simulink model "Wall_Model_Version_1_8_2018a"  (R2018b)
settings: Solver=ode3  StartTime=0.0  StopTime=inf  FixedStep=Ts  RelTol=1e-3  EnableMultiTasking=on
InitFcn:
  | clc;
  | clear all;
  | close all;
  | addpath('D:\Aravind_A0164966M_EE5003\Matlab files\3r2c model')
  | Ts=1
  | Duration=36000;
  | %% Coefficients of Rs and Cs
  | 
  | %% Front Wall
  | l1 = 7.37;
  | b1 = 2.63;
  | y1 = 0.186;
  | x1 = 0.111;
  | y2 = 0.814;
  | x2 = 0.506;
  | x3 = 0.383;
  | 
  | %% Left Wall
  | l2 = 10.11;
  | b2 = 2.63;
  | y3 = 0.186;
  | x4 = 0.111;
  | y4 = 0.814;
  | x5 = 0.506;
  | x6 = 0.383;
  | 
  | %% Left Wall Glass
  | x4_g = 0.5;
  | x5_g = 0.5;
  | y3_g = 1;
  | 
  | %% Right Wall
  | l3 = 7.37;
  | b3 = 2.63;
  | y5 = 0.186;
  | x7 = 0.111;
  | y6 = 0.814;
  | x8 = 0.506;
  | x9 = 0.383;
  | 
  | %% Back Wall
  | l4 = 10.11;
  | b4 = 2.63;
  | y7 = 1;
  | x10 = 0.5;
  | %y8 = 0.5;
  | x11 = 0.5;
  | %x12= 0.33;
  | 
  | %% Roof
  | l5 = 10.11;
  | b5 = 7.37;
  | y9 = 0.186;
  | x13 = 0.111;
  | y10 = 0.814;
  | x14 = 0.506;
  | x15 = 0.383;
  | 
  | %% Floor
  | l6 = 10.11;
  | b6 = 7.37;
  | y11 = 0.186;
  | x16 = 0.111;
  | y12 = 0.814;
  | x17 = 0.506;
  | x18 = 0.383;
  | 
  | %%Areas
  | A1 = l1 * b1;
  | A2 = l2 * b2;
  | A3 = l3 * b3;
  | A4 = l4 * b4;
  | A5 = l5 * b5;
  | A6 = l6 * b6;
  | 
  | %% Initial Temperatures at the surfaces
  | T1_initial_front=301;
  | T2_initial_front=300;
  | 
  | T1_initial_left=301;
  | T2_initial_left=300;
  | 
  | T1_initial_right=301;
  | T2_initial_right=300;
  | 
  | T1_initial_back=301;
  | T2_initial_back=300;
  | 
  | T1_initial_roof=301;
  | T2_initial_roof=300;
  | 
  | T1_initial_floor=301;
  | T2_initial_floor=300;
  | 
  | %ri = 0.1300; % m2 K/W resistance of inner surface of brick wall
  | %rso = 0.04; % m2 K/W resistance of outer surface of the wall
  | 
  | ri = 0;
  | rso = 0;
  | %% Density of Building materials in the room
  | p_conc    = 2400; % kg/m3 density of concrete
  | p_pstr     = 850; % kg/m3 density of plastering
  | p_gb       = 1100; % kg/m3 density of gypsum board
  | p_glass    = 2530; % kg/m3 density of glass
  | p_swood  = 550;   % kg/m3 density of soft-wood
  | 
  | %% Thermal heat capacity of the building materials in the room
  | c_conc    = 840;  % J/kg K heat capacity of concrete
  | c_pstr     = 1000;  %J/kg K heat capacity of plastering
  | c_gb       = 700; % J/kg K heat capacity of gypsum board
  | c_glass    = 840;  % J/kg K heat capacity of glass
  | c_swood  = 1700; % J/kg K heat capacity of soft-wood
  | 
  | %% Thermal conductivity(lamda) of building materials in the room
  | l_conc    = 0.8;  % W/m K Thermal conductivity of concrete
  | l_pstr     = 0.013;  % W/m K Thermal conductivity of plastering
  | l_gb       = 0.35; % W/m K Thermal conductivity of gypsum board
  | l_glass    = 0.8;  % W/m K Thermal conductivity of glass
  | l_swood  = 0.08; % W/m K Thermal conductivity of soft-wood
  | 
  | %% Standard thickness of materials used
  | d_conc = 0.01;  % m Thickness of concrete BCA standard
  | d_pstr = 0.005; % m Thickness of plastering BCA standard
  | d_glass = 0.015; % m Thickness of glass wall widely used
  | d_swood = 0.01; % m Thickness of softwood on the right wall
  | d_gb = 0.015; % m Thickness of gypsum board
  | 
  | %% Resistance and Capacitance of front Wall
  | Rth1 =( ri + rso + (d_conc/l_conc) + (d_pstr/l_pstr))/(A1); % Thermal resistance
  | Cth1 = A1*(d_conc*p_conc*c_conc + d_pstr*p_pstr*c_pstr) ; % Thermal Capacitance
  | 
  | %% Resistance and Capacitance of left Wall concrete
  | A_conc = A2 * 0.5; % Half of the wall on the left is  glass wall
  | Rth2 =( ri + rso + (d_conc/l_conc) + (d_pstr/l_pstr))/(A_conc); % Thermal resistance
  | Cth2 = A_conc*(d_conc*p_conc*c_conc + d_pstr*p_pstr*c_pstr); % Thermal Capacitance
  | 
  | %% Resistance and Capacitance of left Wall glass
  | A_glass = A2 * 0.5; % Half of the wall on the left is  glass wall
  | Rth2_g =(d_glass/l_glass) /(A_glass); % Thermal resistance
  | Cth2_g = A_glass*(d_glass*p_glass*c_glass ); % Thermal Capacitance
  | 
  | %% Resistance and Capacitance of right Wall
  | Rth3 = ( ri + rso+ (d_conc/l_conc) + (d_swood/l_swood))/(A3);% Thermal resistance
  | Cth3 = A3*(d_swood*p_swood*c_swood + d_conc*p_conc*c_conc ); % Thermal Capacitance
  | 
  | %% Resistance and Capacitance of back Wall
  | Rth4 =(d_glass/l_glass) /(A4); % Thermal resistance
  | Cth4 = A4*(d_glass*p_glass*c_glass ); % Thermal Capacitance
  | 
  | %% Resistance and Capacitance of roof Wall
  | Rth5 = (d_gb/l_gb)/(A5);% Thermal resistance
  | Cth5 = A5*(d_gb*p_gb*c_gb ); % Thermal Capacitance
  | 
  | %% Resistance and Capacitance of floor Wall
  | Rth6 = (d_gb/l_gb)/(A6);% Thermal resistance
  | Cth6 = A6*(d_gb*p_gb*c_gb ); % Thermal Capacitance
  | 
  | %% Volume and mass of room
  | density_of_air = 1.184; % kg/m3 at 25 deg. K
  | volume = l1*l2*b1; % m3
  | mass = volume * density_of_air ;% kg
  | specific_heat = 1.005; % J/kg deg.K
  | tic;
  | 
  | Tleft = 298;
libraries: powerlib x70, simulink x1
(part 1 of 2)
settings Model: EnablePacing=on  PacingRate=1000  Creator=elekkr  LastModifiedBy=accma
settings DataIOCC: LimitDataPoints=on  SaveFormat=Array
settings OptimizationCC: LifeSpan=inf
settings DebuggingCC: UnconnectedInputMsg=none  UnconnectedOutputMsg=none  UnconnectedLineMsg=none  LibraryContextMissingDiagnostic=none  SFUnexpectedBacktrackingDiag=warning  SFNoUnconditionalDefaultTransitionDiag=warning  SFExecutionAtInitializationDiag=none
settings HardwareCC: ProdBitPerPointer=32  ProdBitPerSizeT=32  ProdBitPerPtrDiffT=32  ProdLargestAtomicFloat=None  ProdIntDivRoundTo=Undefined  ProdEndianess=Unspecified  ProdWordSize=32  ProdHWDeviceType=32-bit Generic
settings ModelReferenceCC: PropagateSignalLabelsOutOfModel=off
settings SFSimCC: SimUseLocalCustomCode=off
settings RTWCC: RTWUseLocalCustomCode=off
settings CodeAppCC: StateflowObjectComments=on
settings GRTTargetCC: TargetLangStandard=C89/C90 (ANSI)  GeneratePreprocessorConditionals=Disable all
settings ConfigComp: CovMetricSettings=dw  CovHtmlReporting=on  CovSaveCumulativeToWorkspaceVar=on  CovSaveSingleToWorkspaceVar=on  CovExternalEMLEnable=off
settings SimscapeCC: SimscapeNormalizeSystem=off

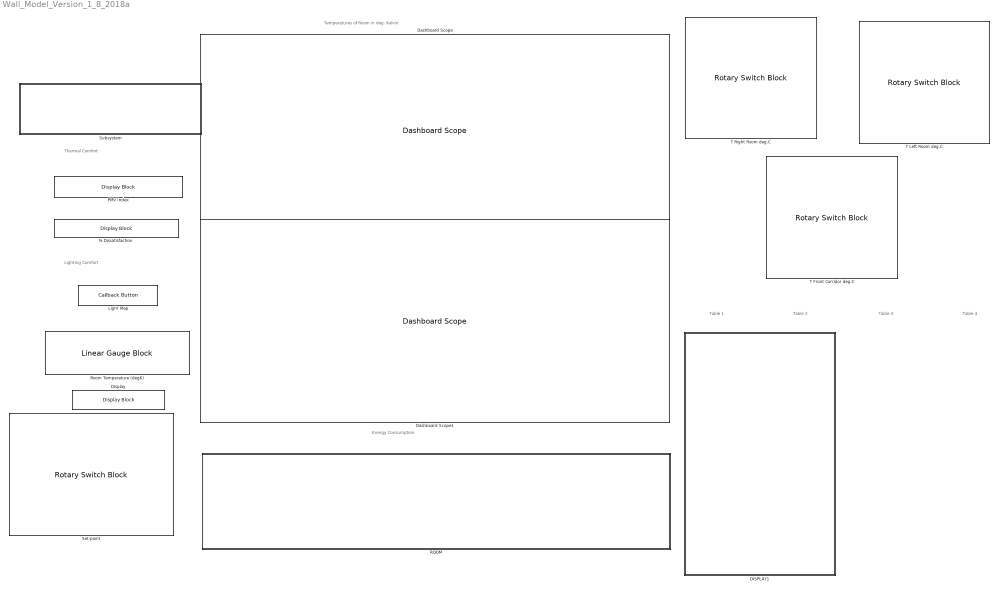
== system Wall_Model_Version_1_8_2018a ==
  note: Table 1
  note: Thermal Comfort
  note: Lighting Comfort
  note: Temperatures of Room in deg. Kelvin
  note: Energy Consumption
  note: Table 2
  note: Table 3
  note: Table 4
  % Dissatisfaction : DisplayBlock  WebBlockId=889  LabelPosition=Hide
  DISPLAY1 : Subsystem  mask(Sensor_node){}
      mask Display: fprintf('CO2 889.35 ppm\n\nCO 1.00 ppm\n\nHCHO 0.03 ppm\n\nO3 0.50 ppm\n\nVOC 0.31 ppm\n\nPM2_5 0.50 ppm\n\nPM10 0.50 ppm\n\nAir Quality Index 82.03\n\n')
  Dashboard Scope : DashboardScope  WebBlockId=1753  Ymin=270  Ymax=330
  Dashboard Scope1 : DashboardScope  WebBlockId=1752  Ymin=0  Ymax=10000
  Display : DisplayBlock  WebBlockId=772  LabelPosition=Hide
  Light Map : CallbackButton  WebBlockId=904
      settings: ClickFcn=heatmap_V2
  PMV Index : DisplayBlock  WebBlockId=888  LabelPosition=Hide
  ROOM : Subsystem
  Room Temperature (degK) : LinearGaugeBlock  WebBlockId=1755  ScaleMin=20  ScaleMax=29  TickInterval=5
  Set-point : RotarySwitchBlock  WebBlockId=542  LabelPosition=Hide
      settings: Values={{'Cold', '', '', 'Optimum', '', '', '', '', '', '', 'Hot'}, [293 294 295 296 297 298 299 300 301 302 303]}
  Subsystem : Subsystem  mask(GBIC_Simulation time){}
      settings: AttributesFormatString=311.25
      mask Display: fprintf('Simulation_Time_Elapsed=1387.00 seconds\nPhysical_Time_Elapsed=311.25 seconds\nSimulation_Speed=4.46 times')
  T Front Corridor deg.C : RotarySwitchBlock  WebBlockId=766  LabelPosition=Hide
      settings: Values={{'20', '21', '22', '23', '24', '25', '26', '27', '28', '29', '30', '31', '32'}, [293 294 295 296 297 298 299 300 301 302 303 304 305]}
  T Left Room deg.C : RotarySwitchBlock  WebBlockId=768  LabelPosition=Hide
      settings: Values={{'20', '21', '22', '23', '24', '25', '26', '27', '28', '29', '30', '31', '32'}, [293 294 295 296 297 298 299 300 301 302 303 304 305]}
  T Right Room deg.C : RotarySwitchBlock  WebBlockId=769  LabelPosition=Hide
      settings: Values={{'20', '21', '22', '23', '24', '25', '26', '27', '28', '29', '30', '31', '32'}, [293 294 295 296 297 298 299 300 301 302 303 304 305]}

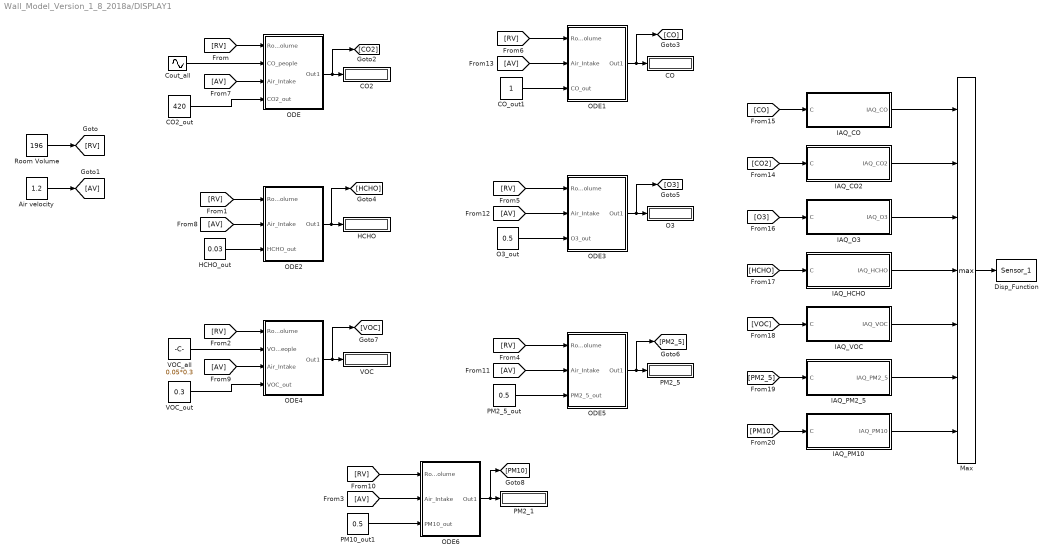
== system Wall_Model_Version_1_8_2018a/DISPLAY1 ==
  Air velocity : Constant  Value=1.2
  CO : Display
  CO2 : Display
  CO2_out : Constant  Value=420
  CO_out1 : Constant
  Cout_all : Sin  Amplitude=150  Bias=550  Frequency=2*pi/(24*3600)
  Disp_Function : M-S-Function  FunctionName=Sensor_1
  HCHO : Display
  HCHO_out : Constant  Value=0.03
  IAQ_CO : MATLAB Function  TreatAsAtomicUnit=on
  IAQ_CO2 : MATLAB Function  TreatAsAtomicUnit=on
  IAQ_HCHO : MATLAB Function  TreatAsAtomicUnit=on
  IAQ_O3 : MATLAB Function  TreatAsAtomicUnit=on
  IAQ_PM10 : MATLAB Function  TreatAsAtomicUnit=on
  IAQ_PM2_5 : MATLAB Function  TreatAsAtomicUnit=on
  IAQ_VOC : MATLAB Function  TreatAsAtomicUnit=on
  Max : MinMax  Function=max  Inputs=7
  O3 : Display
  O3_out : Constant  Value=0.5
  ODE : Subsystem
  ODE1 : Subsystem
  ODE2 : Subsystem
  ODE3 : Subsystem
  ODE4 : Subsystem
  ODE5 : Subsystem
  ODE6 : Subsystem
  PM10_out1 : Constant  Value=0.5
  PM2_1 : Display
  PM2_5 : Display
  PM2_5_out : Constant  Value=0.5
  Room Volume : Constant  Value=196
  VOC : Display
  VOC_all : Constant  Value=0.05*0.3
  VOC_out : Constant  Value=0.3
  wires:
  Cout_all/1 -> ODE/2(CO_people)
  ODE2/1(Out1) -> [HCHO], HCHO/1
  HCHO_out/1 -> ODE2/3(HCHO_out)
  CO_out1/1 -> ODE1/3(CO_out)
  CO2_out/1 -> ODE/4(CO2_out)
  O3_out/1 -> ODE3/3(O3_out)
  ODE3/1(Out1) -> [O3], O3/1
  IAQ_CO/1(IAQ_CO) -> Max/1
  IAQ_HCHO/1(IAQ_HCHO) -> Max/4
  ODE/1(Out1) -> [CO2], CO2/1
  IAQ_CO2/1(IAQ_CO2) -> Max/2
  IAQ_PM2_5/1(IAQ_PM2_5) -> Max/6
  IAQ_VOC/1(IAQ_VOC) -> Max/5
  IAQ_PM10/1(IAQ_PM10) -> Max/7
  ODE1/1(Out1) -> [CO], CO/1
  IAQ_O3/1(IAQ_O3) -> Max/3
  ODE5/1(Out1) -> [PM2_5], PM2_5/1
  PM2_5_out/1 -> ODE5/3(PM2_5_out)
  Room Volume/1 -> [RV]
  [RV] -> ODE/1(Room_Volume)
  [RV] -> ODE2/1(Room_Volume)
  [RV] -> ODE5/1(Room_Volume)
  [RV] -> ODE3/1(Room_Volume)
  [RV] -> ODE1/1(Room_Volume)
  Air velocity/1 -> [AV]
  [AV] -> ODE/3(Air_Intake)
  [AV] -> ODE2/2(Air_Intake)
  [AV] -> ODE5/2(Air_Intake)
  [AV] -> ODE3/2(Air_Intake)
  [AV] -> ODE1/2(Air_Intake)
  [RV] -> ODE4/1(Room_Volume)
  ODE4/1(Out1) -> [VOC], VOC/1
  [AV] -> ODE4/3(Air_Intake)
  VOC_out/1 -> ODE4/4(VOC_out)
  VOC_all/1 -> ODE4/2(VOC_people)
  [AV] -> ODE6/2(Air_Intake)
  [RV] -> ODE6/1(Room_Volume)
  PM10_out1/1 -> ODE6/3(PM10_out)
  [CO2] -> IAQ_CO2/1(C)
  [CO] -> IAQ_CO/1(C)
  [O3] -> IAQ_O3/1(C)
  [HCHO] -> IAQ_HCHO/1(C)
  [VOC] -> IAQ_VOC/1(C)
  [PM2_5] -> IAQ_PM2_5/1(C)
  [PM10] -> IAQ_PM10/1(C)
  ODE6/1(Out1) -> [PM10], PM2_1/1
  Max/1 -> Disp_Function/1

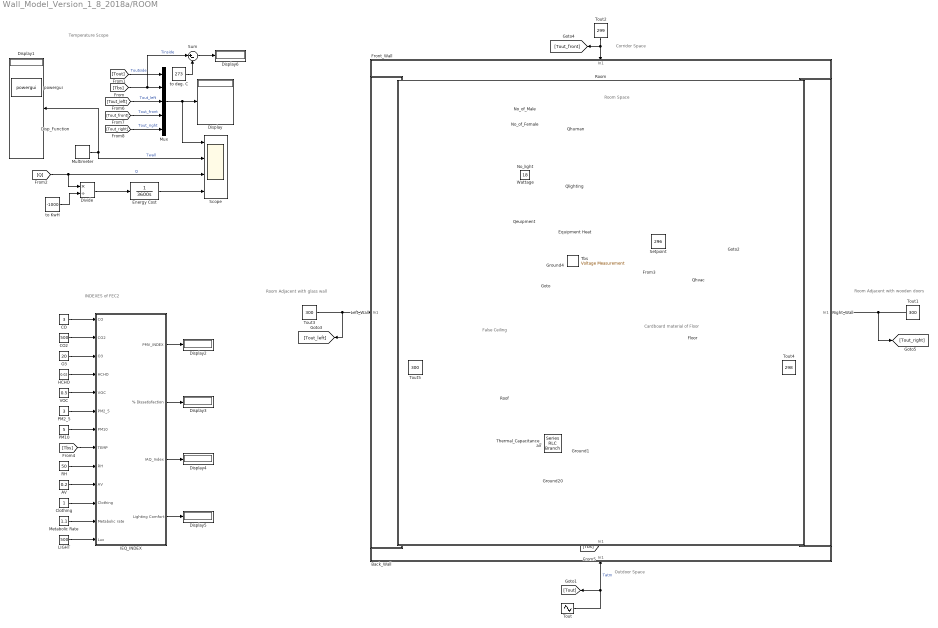
== system Wall_Model_Version_1_8_2018a/ROOM ==
  note: INDEXES of FEC2
  note: False Ceiling
  note: Cardboard material of Floor
  note: Room Adjacent with wooden doors
  note: Corridor Space
  note: Room Adjacent with glass wall
  note: Outdoor Space
  note: Room Space
  note: Temperature Scope
  AV : Constant  Value=0.2
  Back_Wall : Subsystem
      mask Display: fprintf('Temperature Outside= 30.30 deg. C\n')
  CO : Constant  Value=3
  CO2 : Constant  Value=500
  Clothing : Constant
  Disp_Function : M-S-Function  FunctionName=fn_IEQ
  Display{,1..6} (7 alike) : Display
  Divide : Product  Inputs=*/
  Energy Cost : TransferFcn  Denominator=[3600 0]
  Equipment Heat : Subsystem
  Floor : Subsystem
      mask Display: fprintf('Temperature \n Below= \n25.00 deg. C\n')
  Front_Wall : Subsystem
      mask Display: fprintf('Temperature Corridor= 26.00 deg. C\n')
  Ground1 : powerlib/Elements/Ground  LConnTagsString=a
      settings: SourceProductName=Simscape Electrical
  Ground20 : powerlib/Elements/Ground  LConnTagsString=a
      settings: SourceProductName=Simscape Electrical
  Ground4 : powerlib/Elements/Ground  LConnTagsString=a
      settings: SourceProductName=Simscape Electrical
  HCHO : Constant  Value=0.02
  IEQ_INDEX : Subsystem
  LIGHT : Constant  Value=500
  Left_Wall : Subsystem
      mask Display: fprintf('Temperature \n Left Room= \n27.00 deg. C\n')
  Metabolic Rate : Constant  Value=1.1
  Multimeter : powerlib/Measurements/Multimeter  PhasorSimulation=off  OutputType=Complex  sel=1  L=12  Gain=0  yselected={}  PSBOutputType=1  PSBequivalent=0  AxesSetting=[0,0.1,-100,100]  Display=0  SavedBlockNames=-11
      settings: SourceProductName=Simscape Electrical
  Mux : Mux  Inputs=5
  No_light : Constant  Value=60
  No_of_Female : Constant  Value=8
  No_of_Male : Constant  Value=8
  O3 : Constant  Value=20
  PM10 : Constant  Value=5
  PM2_5 : Constant  Value=3
  Qeuipment : Sin  Amplitude=200  Bias=3200  Frequency=2*pi/(12*3600)  SampleTime=0
  Qhuman : Subsystem
  Qhvac : Subsystem
  Qlighting : Subsystem
  RH : Constant  Value=50
  Right_Wall : Subsystem
      mask Display: fprintf('Temperature \n Right Room= \n27.00 deg. C\n')
  Roof : Subsystem
      mask Display: fprintf('Temperature \n Above Roof= \n27.00 deg. C\n')
  Room : Subsystem
      mask Display: fprintf('Temperature Room= 23.00 deg. C\n')
  Scope : Scope  NumInputPorts=4
  Setpoint : Constant  Value=296
  Sum : Sum  Inputs=|+-
  Tbs : powerlib/Measurements/Voltage Measurement  PhasorSimulation=off  OutputType=Magnitude  PSBequivalent=0
      settings: SourceProductName=Simscape Electrical
  Thermal_Capacitance_air : powerlib/Elements/Series RLC Branch  LConnTagsString=__new0  RConnTagsString=__new0  BranchType=C  Resistance=0  Inductance=1e-3  SetiL0=off  InitialCurrent=0  Capacitance=density_of_air * volume * specific_heat  Setx0=on  InitialVoltage=298  Measurements=Branch voltage
      settings: SourceProductName=Simscape Electrical
  Tout : Sin  Amplitude=1.5  Bias=303  Frequency=2*pi/(12*3600)
  Tout1 : Constant  Value=300
  Tout2 : Constant  Value=299
  Tout3 : Constant  Value=300
  Tout4 : Constant  Value=298
  Tout5 : Constant  Value=300
  VOC : Constant  Value=0.5
  Wattage : Constant  Value=18
  powergui : powerlib/powergui  Priority=1  SimulationMode=Discrete  SampleTime=Ts  frequency=60  Iterations=50  frequencyindice=0  Pbase=100e6  ErrMax=1e-4  UnitsV=kV  UnitsW=MW  buscounter=0  FunctionMessages=off  echomessages=off  EnableUseOfTLC=off  CurrentSourceSwitches=off  DisableSnubberDevices=off  DisableRonSwitches=off  DisableVfSwitches=off  DisplayEquations=off  SolverType=Tustin/Backward Euler (TBE)  Interpol=off  ExternalGateDelay=off  methode=off  Ts=100  x0status=blocks  SPID=off  SwTol=0  HookPort=off  RestoreLinks=warning  ResistiveCurrentMeasurement=off  Frange=[0:2:500]  Ylog=off  Xlog=on  ShowGrid=off  save=off  variable=ZData  structure=0  ZoomFFT=off  StartTime=0.0  cycles=1  DisplayStyle=1  fundamental=60  FreqAxis=off  MaxFrequency=1000  frequencyindicesteady=1  RmsSteady=1  display=off
      settings: SourceProductName=Simscape Electrical
  to KwH : Constant  Value=-1000
  to deg. C : Constant  Value=273
  wires:
  No_of_Female/1 -> Qhuman/2(No_Female)
  Tout5/1 -> Roof/1(In1)
  Tout3/1 -> [Tout_left], Left_Wall/1(In1)
  [Tout] -> Mux/1  "Toutside"
  [Q] -> Scope/3, Divide/1  "Q"
  Setpoint/1 -> Qhvac/1(Setpoint)
  Qhvac/1(Qhvac) -> [Q]
  Tout1/1 -> [Tout_right], Right_Wall/1(In1)
  Tout/1 -> [Tout], Back_Wall/1(In1)  "Tatm"
  Tout4/1 -> Floor/1(In1)
  [Tout_front] -> Mux/4  "Tout_front"
  No_light/1 -> Qlighting/1("No_light ")
  Tout2/1 -> [Tout_front], Front_Wall/1(In1)
  Multimeter/1 -> Scope/2, Display1/1  "Twall"
  [Tout_right] -> Mux/5  "Tout_right"
  [Tout_left] -> Mux/3  "Tout_left"
  No_of_Male/1 -> Qhuman/1("No_Male ")
  Wattage/1 -> Qlighting/2(Wattage)
  Mux/1 -> Scope/1, Display/1
  Qeuipment/1 -> Equipment Heat/1(In1)
  to KwH/1 -> Divide/2
  Energy Cost/1 -> Scope/4
  Divide/1 -> Energy Cost/1
  [Tbs] -> IEQ_INDEX/8(TEMP)
  CO/1 -> IEQ_INDEX/1(CO)
  PM10/1 -> IEQ_INDEX/7(PM10)
  PM2_5/1 -> IEQ_INDEX/6(PM2_5)
  VOC/1 -> IEQ_INDEX/5(VOC)
  HCHO/1 -> IEQ_INDEX/4(HCHO)
  O3/1 -> IEQ_INDEX/3(O3)
  CO2/1 -> IEQ_INDEX/2(CO2)
  RH/1 -> IEQ_INDEX/9(RH)
  AV/1 -> IEQ_INDEX/10(AV)
  Clothing/1 -> IEQ_INDEX/11(Clothing)
  IEQ_INDEX/1(PMV_INDEX) -> Display2/1
  IEQ_INDEX/2("% Dissatisfaction ") -> Display3/1
  LIGHT/1 -> IEQ_INDEX/13(Lux)
  Metabolic Rate/1 -> IEQ_INDEX/12(Metabolic rate)
  IEQ_INDEX/3(IAQ_Index) -> Display4/1
  IEQ_INDEX/4(Lighting Comfort) -> Display5/1
  Tbs/1 -> [Tbs]
  [Tbs] -> Sum/1, Mux/2  "Tinside"
  [Tbs] -> Qhvac/2(Tbs)
  [Tbs] -> Room/1(In1)
  to deg. C/1 -> Sum/2
  Sum/1 -> Display6/1
  connections:
  Ground4/LConn1 -- Tbs/LConn2
  Equipment Heat/RConn1 -- Qhvac/RConn1 -- Right_Wall/RConn1 -- Roof/RConn1 -- Back_Wall/RConn1 -- Floor/RConn1 -- Left_Wall/RConn1 -- Tbs/LConn1 -- Qlighting/RConn1 -- Qhuman/RConn1 -- Front_Wall/RConn1
  Ground20/LConn1 -- Thermal_Capacitance_air/RConn1
  Thermal_Capacitance_air/LConn1 -- Ground1/LConn1

== system Wall_Model_Version_1_8_2018a/Subsystem ==
  Disp_Function : M-S-Function  FunctionName=fn_Display

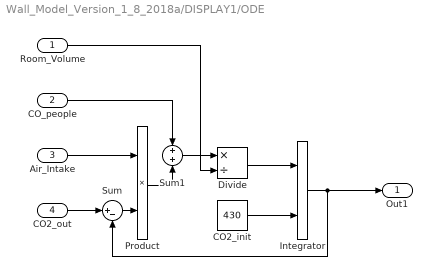
== system Wall_Model_Version_1_8_2018a/DISPLAY1/ODE ==
  Room_Volume : Inport
  CO_people : Inport  Port=2
  Air_Intake : Inport  Port=3
  CO2_out : Inport  Port=4
  CO2_init : Constant  Value=430
  Divide : Product  Inputs=*/
  Integrator : Integrator  InitialConditionSource=external
  Product : Product
  Sum : Sum  Inputs=|+-
  Sum1 : Sum
  Out1 : Outport
  wires:
  Air_Intake/1 -> Product/1
  Room_Volume/1 -> Divide/2
  Product/1 -> Sum1/2
  CO2_out/1 -> Sum/1
  Integrator/1 -> Sum/2, Out1/1
  Sum/1 -> Product/2
  CO2_init/1 -> Integrator/2
  CO_people/1 -> Sum1/1
  Divide/1 -> Integrator/1
  Sum1/1 -> Divide/1

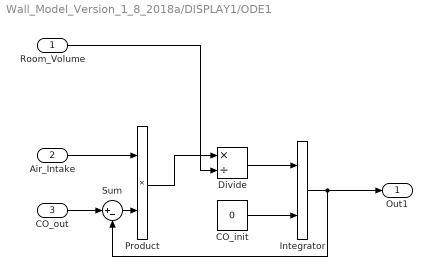
== system Wall_Model_Version_1_8_2018a/DISPLAY1/ODE1 ==
  Room_Volume : Inport
  Air_Intake : Inport  Port=2
  CO_out : Inport  Port=3
  CO_init : Constant  Value=0
  Divide : Product  Inputs=*/
  Integrator : Integrator  InitialConditionSource=external
  Product : Product
  Sum : Sum  Inputs=|+-
  Out1 : Outport
  wires:
  Air_Intake/1 -> Product/1
  Room_Volume/1 -> Divide/2
  CO_out/1 -> Sum/1
  Integrator/1 -> Sum/2, Out1/1
  Sum/1 -> Product/2
  CO_init/1 -> Integrator/2
  Divide/1 -> Integrator/1
  Product/1 -> Divide/1

== system Wall_Model_Version_1_8_2018a/DISPLAY1/ODE2 ==
  Room_Volume : Inport
  Air_Intake : Inport  Port=2
  HCHO_out : Inport  Port=3
  Divide : Product  Inputs=*/
  HCHO_init : Constant  Value=0
  Integrator : Integrator  InitialConditionSource=external
  Product : Product
  Sum : Sum  Inputs=|+-
  Out1 : Outport
  wires:
  Air_Intake/1 -> Product/1
  Room_Volume/1 -> Divide/2
  HCHO_out/1 -> Sum/1
  Integrator/1 -> Sum/2, Out1/1
  Sum/1 -> Product/2
  HCHO_init/1 -> Integrator/2
  Divide/1 -> Integrator/1
  Product/1 -> Divide/1

== system Wall_Model_Version_1_8_2018a/DISPLAY1/ODE3 ==
  Room_Volume : Inport
  Air_Intake : Inport  Port=2
  O3_out : Inport  Port=3
  Divide : Product  Inputs=*/
  Integrator : Integrator  InitialConditionSource=external
  O3_init : Constant  Value=0
  Product : Product
  Sum : Sum  Inputs=|+-
  Out1 : Outport
  wires:
  Air_Intake/1 -> Product/1
  Room_Volume/1 -> Divide/2
  O3_out/1 -> Sum/1
  Integrator/1 -> Sum/2, Out1/1
  Sum/1 -> Product/2
  O3_init/1 -> Integrator/2
  Divide/1 -> Integrator/1
  Product/1 -> Divide/1

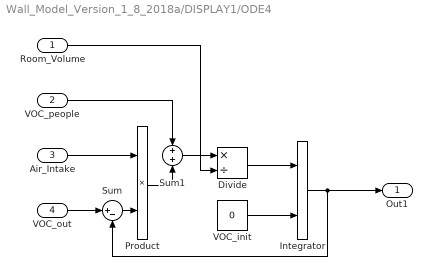
== system Wall_Model_Version_1_8_2018a/DISPLAY1/ODE4 ==
  Room_Volume : Inport
  VOC_people : Inport  Port=2
  Air_Intake : Inport  Port=3
  VOC_out : Inport  Port=4
  Divide : Product  Inputs=*/
  Integrator : Integrator  InitialConditionSource=external
  Product : Product
  Sum : Sum  Inputs=|+-
  Sum1 : Sum
  VOC_init : Constant  Value=0
  Out1 : Outport
  wires:
  Air_Intake/1 -> Product/1
  Room_Volume/1 -> Divide/2
  Product/1 -> Sum1/2
  VOC_out/1 -> Sum/1
  Integrator/1 -> Sum/2, Out1/1
  Sum/1 -> Product/2
  VOC_init/1 -> Integrator/2
  VOC_people/1 -> Sum1/1
  Divide/1 -> Integrator/1
  Sum1/1 -> Divide/1

== system Wall_Model_Version_1_8_2018a/DISPLAY1/ODE5 ==
  Room_Volume : Inport
  Air_Intake : Inport  Port=2
  PM2_5_out : Inport  Port=3
  Divide : Product  Inputs=*/
  Integrator : Integrator  InitialConditionSource=external
  PM2_5_init : Constant  Value=0
  Product : Product
  Sum : Sum  Inputs=|+-
  Out1 : Outport
  wires:
  Air_Intake/1 -> Product/1
  Room_Volume/1 -> Divide/2
  PM2_5_out/1 -> Sum/1
  Integrator/1 -> Sum/2, Out1/1
  Sum/1 -> Product/2
  PM2_5_init/1 -> Integrator/2
  Divide/1 -> Integrator/1
  Product/1 -> Divide/1

== system Wall_Model_Version_1_8_2018a/DISPLAY1/ODE6 ==
  Room_Volume : Inport
  Air_Intake : Inport  Port=2
  PM10_out : Inport  Port=3
  Divide : Product  Inputs=*/
  Integrator : Integrator  InitialConditionSource=external
  PM10_init : Constant  Value=0
  Product : Product
  Sum : Sum  Inputs=|+-
  Out1 : Outport
  wires:
  Product/1 -> Divide/1
  Divide/1 -> Integrator/1
  PM10_init/1 -> Integrator/2
  Sum/1 -> Product/2
  Integrator/1 -> Out1/1, Sum/2
  PM10_out/1 -> Sum/1
  Room_Volume/1 -> Divide/2
  Air_Intake/1 -> Product/1

== system Wall_Model_Version_1_8_2018a/ROOM/Back_Wall ==
  note: T1
  note: Back Wall
  In1 : Inport
  Disp_Function : M-S-Function  FunctionName=fn_Display_wall
  Ground1 : powerlib/Elements/Ground  LConnTagsString=a
      settings: SourceProductName=Simscape Electrical
  Ground2 : powerlib/Elements/Ground  LConnTagsString=a
      settings: SourceProductName=Simscape Electrical
  V : powerlib/Electrical Sources/Controlled Voltage Source  Initialize=on  Source_Type=AC  Amplitude=0  Phase=0  Frequency=0  Measurements=None
      settings: SourceProductName=Simscape Electrical
  x10*Rth4 : powerlib/Elements/Series RLC Branch  LConnTagsString=__new0  RConnTagsString=__new0  BranchType=R  Resistance=x10*Rth4  Inductance=1e-3  SetiL0=off  InitialCurrent=0  Capacitance=1e-6  Setx0=off  InitialVoltage=0  Measurements=None
      settings: SourceProductName=Simscape Electrical
  x11*Rth4 : powerlib/Elements/Series RLC Branch  LConnTagsString=__new0  RConnTagsString=__new0  BranchType=R  Resistance=x11*Rth4  Inductance=1e-3  SetiL0=off  InitialCurrent=0  Capacitance=1e-6  Setx0=off  InitialVoltage=0  Measurements=None
      settings: SourceProductName=Simscape Electrical
  y7*Cth4 : powerlib/Elements/Series RLC Branch  LConnTagsString=__new0  RConnTagsString=__new0  BranchType=C  Resistance=0  Inductance=1e-3  SetiL0=off  InitialCurrent=0  Capacitance=y7*Cth4  Setx0=on  InitialVoltage=T1_initial_back  Measurements=Branch voltage
      settings: SourceProductName=Simscape Electrical
  Conn1 : PMIOPort  Side=Right
  wires:
  In1/1 -> Disp_Function/1, V/1
  connections:
  Ground2/LConn1 -- V/LConn1
  V/RConn1 -- x10*Rth4/LConn1
  x10*Rth4/RConn1 -- y7*Cth4/LConn1 -- x11*Rth4/LConn1
  Ground1/LConn1 -- y7*Cth4/RConn1
  x11*Rth4/RConn1 -- Conn1/RConn1

== system Wall_Model_Version_1_8_2018a/ROOM/Equipment Heat ==
  In1 : Inport
  Ground20 : powerlib/Elements/Ground  LConnTagsString=a
      settings: SourceProductName=Simscape Electrical
  I1 : powerlib/Electrical Sources/Controlled Current Source  Initialize=off  Source_Type=AC  Amplitude=1  Phase=0  Frequency=0  Measurements=None
      settings: SourceProductName=Simscape Electrical
  Conn1 : PMIOPort  Side=Right
  wires:
  In1/1 -> I1/1
  connections:
  Ground20/LConn1 -- I1/LConn1
  I1/RConn1 -- Conn1/RConn1

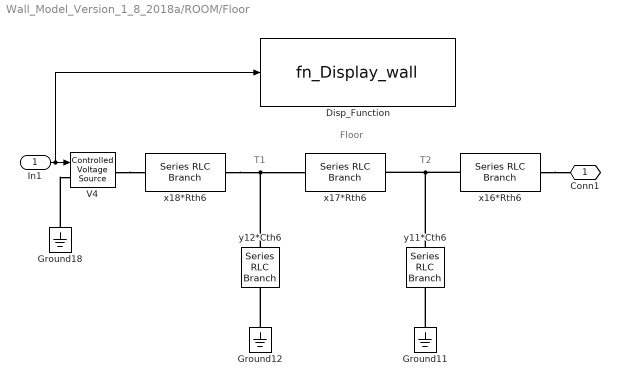
== system Wall_Model_Version_1_8_2018a/ROOM/Floor ==
  note: T2
  note: T1
  note: Floor
  In1 : Inport
  Disp_Function : M-S-Function  FunctionName=fn_Display_wall
  Ground11 : powerlib/Elements/Ground  LConnTagsString=a
      settings: SourceProductName=Simscape Electrical
  Ground12 : powerlib/Elements/Ground  LConnTagsString=a
      settings: SourceProductName=Simscape Electrical
  Ground18 : powerlib/Elements/Ground  LConnTagsString=a
      settings: SourceProductName=Simscape Electrical
  V4 : powerlib/Electrical Sources/Controlled Voltage Source  Initialize=on  Source_Type=AC  Amplitude=0  Phase=0  Frequency=0  Measurements=None
      settings: SourceProductName=Simscape Electrical
  x16*Rth6 : powerlib/Elements/Series RLC Branch  LConnTagsString=__new0  RConnTagsString=__new0  BranchType=R  Resistance=x16*Rth6  Inductance=1e-3  SetiL0=off  InitialCurrent=0  Capacitance=1e-6  Setx0=off  InitialVoltage=0  Measurements=None
      settings: SourceProductName=Simscape Electrical
  x17*Rth6 : powerlib/Elements/Series RLC Branch  LConnTagsString=__new0  RConnTagsString=__new0  BranchType=R  Resistance=x17*Rth6  Inductance=1e-3  SetiL0=off  InitialCurrent=0  Capacitance=1e-6  Setx0=off  InitialVoltage=0  Measurements=None
      settings: SourceProductName=Simscape Electrical
  x18*Rth6 : powerlib/Elements/Series RLC Branch  LConnTagsString=__new0  RConnTagsString=__new0  BranchType=R  Resistance=x18*Rth6  Inductance=1e-3  SetiL0=off  InitialCurrent=0  Capacitance=1e-6  Setx0=off  InitialVoltage=0  Measurements=None
      settings: SourceProductName=Simscape Electrical
  y11*Cth6 : powerlib/Elements/Series RLC Branch  LConnTagsString=__new0  RConnTagsString=__new0  BranchType=C  Resistance=0  Inductance=1e-3  SetiL0=off  InitialCurrent=0  Capacitance=y11*Cth6  Setx0=on  InitialVoltage=T1_initial_floor  Measurements=Branch voltage
      settings: SourceProductName=Simscape Electrical
  y12*Cth6 : powerlib/Elements/Series RLC Branch  LConnTagsString=__new0  RConnTagsString=__new0  BranchType=C  Resistance=0  Inductance=1e-3  SetiL0=off  InitialCurrent=0  Capacitance=y12*Cth6  Setx0=on  InitialVoltage=T2_initial_floor  Measurements=Branch voltage
      settings: SourceProductName=Simscape Electrical
  Conn1 : PMIOPort  Side=Right
  wires:
  In1/1 -> Disp_Function/1, V4/1
  connections:
  V4/RConn1 -- x18*Rth6/LConn1
  y11*Cth6/LConn1 -- x16*Rth6/LConn1 -- x17*Rth6/RConn1
  y12*Cth6/LConn1 -- x18*Rth6/RConn1 -- x17*Rth6/LConn1
  Ground18/LConn1 -- V4/LConn1
  Ground11/LConn1 -- y11*Cth6/RConn1
  Ground12/LConn1 -- y12*Cth6/RConn1
  x16*Rth6/RConn1 -- Conn1/RConn1

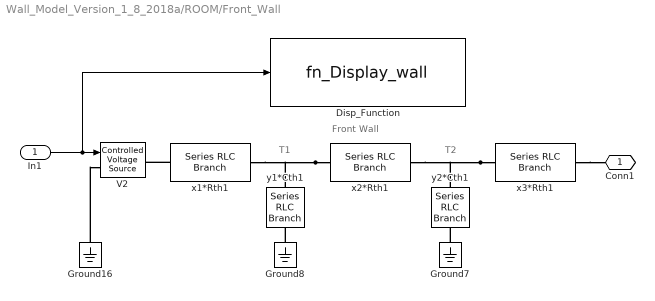
== system Wall_Model_Version_1_8_2018a/ROOM/Front_Wall ==
  note: Front Wall
  note: T2
  note: T1
  In1 : Inport
  Disp_Function : M-S-Function  FunctionName=fn_Display_wall
  Ground16 : powerlib/Elements/Ground  LConnTagsString=a
      settings: SourceProductName=Simscape Electrical
  Ground7 : powerlib/Elements/Ground  LConnTagsString=a
      settings: SourceProductName=Simscape Electrical
  Ground8 : powerlib/Elements/Ground  LConnTagsString=a
      settings: SourceProductName=Simscape Electrical
  V2 : powerlib/Electrical Sources/Controlled Voltage Source  Initialize=on  Source_Type=AC  Amplitude=0  Phase=0  Frequency=0  Measurements=None
      settings: SourceProductName=Simscape Electrical
  x1*Rth1 : powerlib/Elements/Series RLC Branch  LConnTagsString=__new0  RConnTagsString=__new0  BranchType=R  Resistance=x1*Rth1  Inductance=1e-3  SetiL0=off  InitialCurrent=0  Capacitance=1e-6  Setx0=off  InitialVoltage=0  Measurements=None
      settings: SourceProductName=Simscape Electrical
  x2*Rth1 : powerlib/Elements/Series RLC Branch  LConnTagsString=__new0  RConnTagsString=__new0  BranchType=R  Resistance=x2*Rth1  Inductance=1e-3  SetiL0=off  InitialCurrent=0  Capacitance=1e-6  Setx0=off  InitialVoltage=0  Measurements=None
      settings: SourceProductName=Simscape Electrical
  x3*Rth1 : powerlib/Elements/Series RLC Branch  LConnTagsString=__new0  RConnTagsString=__new0  BranchType=R  Resistance=x3*Rth1  Inductance=1e-3  SetiL0=off  InitialCurrent=0  Capacitance=1e-6  Setx0=off  InitialVoltage=0  Measurements=None
      settings: SourceProductName=Simscape Electrical
  y1*Cth1 : powerlib/Elements/Series RLC Branch  LConnTagsString=__new0  RConnTagsString=__new0  BranchType=C  Resistance=0  Inductance=1e-3  SetiL0=off  InitialCurrent=0  Capacitance=y1*Cth1  Setx0=on  InitialVoltage=T1_initial_front  Measurements=Branch voltage
      settings: SourceProductName=Simscape Electrical
  y2*Cth1 : powerlib/Elements/Series RLC Branch  LConnTagsString=__new0  RConnTagsString=__new0  BranchType=C  Resistance=0  Inductance=1e-3  SetiL0=off  InitialCurrent=0  Capacitance=y2*Cth1  Setx0=on  InitialVoltage=T2_initial_front  Measurements=Branch voltage
      settings: SourceProductName=Simscape Electrical
  Conn1 : PMIOPort  Side=Right
  wires:
  In1/1 -> Disp_Function/1, V2/1
  connections:
  Ground7/LConn1 -- y2*Cth1/RConn1
  x2*Rth1/LConn1 -- x1*Rth1/RConn1 -- y1*Cth1/LConn1
  x3*Rth1/LConn1 -- x2*Rth1/RConn1 -- y2*Cth1/LConn1
  Ground16/LConn1 -- V2/LConn1
  Ground8/LConn1 -- y1*Cth1/RConn1
  x1*Rth1/LConn1 -- V2/RConn1
  x3*Rth1/RConn1 -- Conn1/RConn1

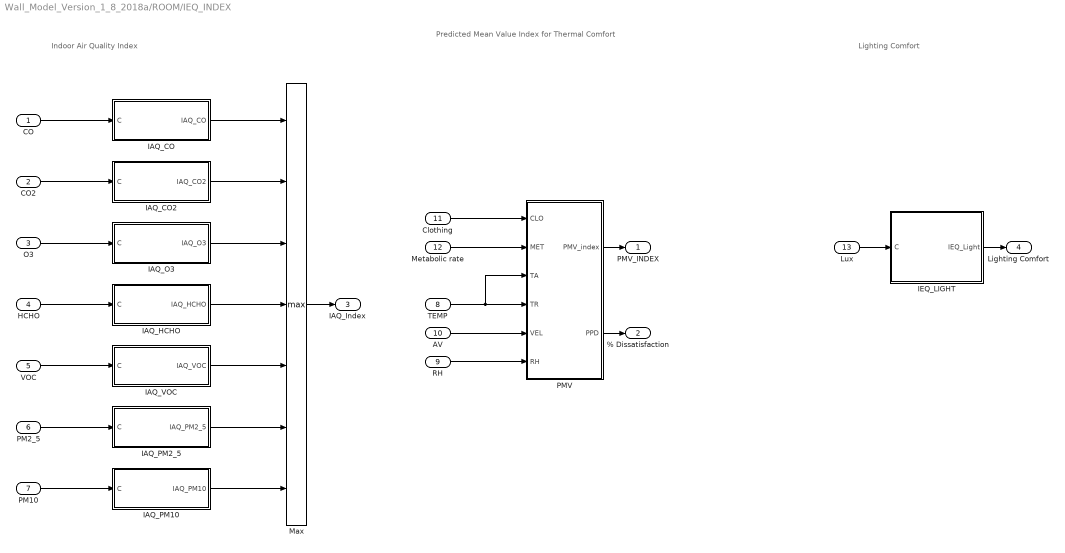
== system Wall_Model_Version_1_8_2018a/ROOM/IEQ_INDEX ==
  note: Indoor Air Quality Index
  note: Predicted Mean Value Index
      | for Thermal Comfort
  note: Lighting Comfort
  CO : Inport
  CO2 : Inport  Port=2
  O3 : Inport  Port=3
  HCHO : Inport  Port=4
  VOC : Inport  Port=5
  PM2_5 : Inport  Port=6
  PM10 : Inport  Port=7
  TEMP : Inport  Port=8
  RH : Inport  Port=9
  AV : Inport  Port=10
  Clothing : Inport  Port=11
  Metabolic rate : Inport  Port=12
  Lux : Inport  Port=13
  IAQ_CO : MATLAB Function  TreatAsAtomicUnit=on
  IAQ_CO2 : MATLAB Function  TreatAsAtomicUnit=on
  IAQ_HCHO : MATLAB Function  TreatAsAtomicUnit=on
  IAQ_O3 : MATLAB Function  TreatAsAtomicUnit=on
  IAQ_PM10 : MATLAB Function  TreatAsAtomicUnit=on
  IAQ_PM2_5 : MATLAB Function  TreatAsAtomicUnit=on
  IAQ_VOC : MATLAB Function  TreatAsAtomicUnit=on
  IEQ_LIGHT : MATLAB Function  TreatAsAtomicUnit=on
  Max : MinMax  Function=max  Inputs=7
  PMV : MATLAB Function  TreatAsAtomicUnit=on
  PMV_INDEX : Outport
  "% Dissatisfaction " : Outport  Port=2
  IAQ_Index : Outport  Port=3
  Lighting Comfort : Outport  Port=4
  wires:
  CO/1 -> IAQ_CO/1(C)
  IAQ_PM10/1(IAQ_PM10) -> Max/7
  IAQ_VOC/1(IAQ_VOC) -> Max/5
  CO2/1 -> IAQ_CO2/1(C)
  PM2_5/1 -> IAQ_PM2_5/1(C)
  IAQ_CO/1(IAQ_CO) -> Max/1
  PM10/1 -> IAQ_PM10/1(C)
  IAQ_PM2_5/1(IAQ_PM2_5) -> Max/6
  IAQ_HCHO/1(IAQ_HCHO) -> Max/4
  IAQ_CO2/1(IAQ_CO2) -> Max/2
  HCHO/1 -> IAQ_HCHO/1(C)
  VOC/1 -> IAQ_VOC/1(C)
  IAQ_O3/1(IAQ_O3) -> Max/3
  O3/1 -> IAQ_O3/1(C)
  RH/1 -> PMV/6(RH)
  AV/1 -> PMV/5(VEL)
  TEMP/1 -> PMV/3(TA), PMV/4(TR)
  Metabolic rate/1 -> PMV/2(MET)
  Clothing/1 -> PMV/1(CLO)
  PMV/1(PMV_index) -> PMV_INDEX/1
  PMV/2(PPD) -> "% Dissatisfaction "/1
  Max/1 -> IAQ_Index/1
  Lux/1 -> IEQ_LIGHT/1(C)
  IEQ_LIGHT/1(IEQ_Light) -> Lighting Comfort/1

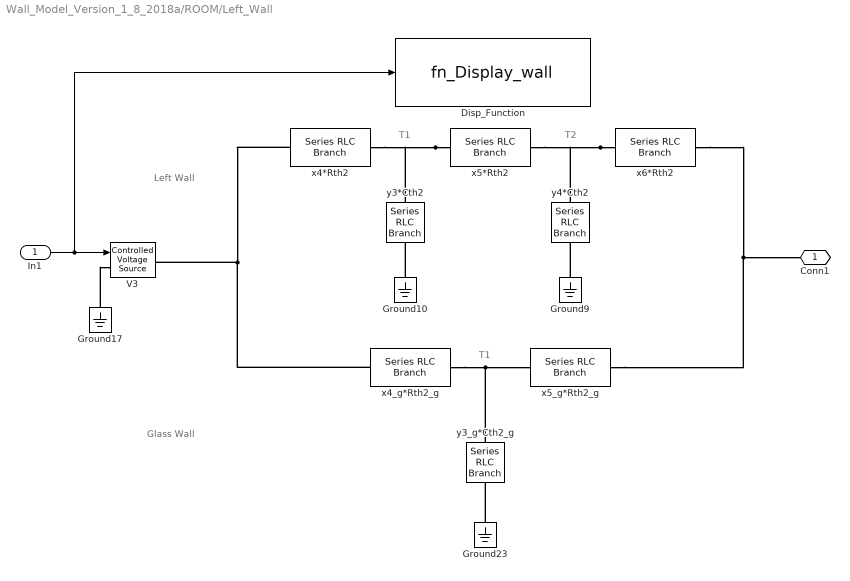
== system Wall_Model_Version_1_8_2018a/ROOM/Left_Wall ==
  note: T1
  note: Glass Wall
  note: Left Wall
  note: T2
  note: T1
  In1 : Inport
  Disp_Function : M-S-Function  FunctionName=fn_Display_wall
  Ground{9..10,17,23} (4 alike) : powerlib/Elements/Ground  LConnTagsString=a
      settings: SourceProductName=Simscape Electrical
  V3 : powerlib/Electrical Sources/Controlled Voltage Source  Initialize=on  Source_Type=AC  Amplitude=0  Phase=0  Frequency=0  Measurements=None
      settings: SourceProductName=Simscape Electrical
  x4*Rth2 : powerlib/Elements/Series RLC Branch  LConnTagsString=__new0  RConnTagsString=__new0  BranchType=R  Resistance=x4*Rth2  Inductance=1e-3  SetiL0=off  InitialCurrent=0  Capacitance=1e-6  Setx0=off  InitialVoltage=0  Measurements=None
      settings: SourceProductName=Simscape Electrical
  x4_g*Rth2_g : powerlib/Elements/Series RLC Branch  LConnTagsString=__new0  RConnTagsString=__new0  BranchType=R  Resistance=x4_g*Rth2_g  Inductance=1e-3  SetiL0=off  InitialCurrent=0  Capacitance=1e-6  Setx0=off  InitialVoltage=0  Measurements=None
      settings: SourceProductName=Simscape Electrical
  x5*Rth2 : powerlib/Elements/Series RLC Branch  LConnTagsString=__new0  RConnTagsString=__new0  BranchType=R  Resistance=x5*Rth2  Inductance=1e-3  SetiL0=off  InitialCurrent=0  Capacitance=1e-6  Setx0=off  InitialVoltage=0  Measurements=None
      settings: SourceProductName=Simscape Electrical
  x5_g*Rth2_g : powerlib/Elements/Series RLC Branch  LConnTagsString=__new0  RConnTagsString=__new0  BranchType=R  Resistance=x5_g*Rth2_g  Inductance=1e-3  SetiL0=off  InitialCurrent=0  Capacitance=1e-6  Setx0=off  InitialVoltage=0  Measurements=None
      settings: SourceProductName=Simscape Electrical
  x6*Rth2 : powerlib/Elements/Series RLC Branch  LConnTagsString=__new0  RConnTagsString=__new0  BranchType=R  Resistance=x6*Rth2  Inductance=1e-3  SetiL0=off  InitialCurrent=0  Capacitance=1e-6  Setx0=off  InitialVoltage=0  Measurements=None
      settings: SourceProductName=Simscape Electrical
  y3*Cth2 : powerlib/Elements/Series RLC Branch  LConnTagsString=__new0  RConnTagsString=__new0  BranchType=C  Resistance=0  Inductance=1e-3  SetiL0=off  InitialCurrent=0  Capacitance=y3*Cth2  Setx0=on  InitialVoltage=T1_initial_left  Measurements=Branch voltage
      settings: SourceProductName=Simscape Electrical
  y3_g*Cth2_g : powerlib/Elements/Series RLC Branch  LConnTagsString=__new0  RConnTagsString=__new0  BranchType=C  Resistance=0  Inductance=1e-3  SetiL0=off  InitialCurrent=0  Capacitance=y3_g*Cth2_g  Setx0=on  InitialVoltage=T1_initial_left  Measurements=Branch voltage
      settings: SourceProductName=Simscape Electrical
  y4*Cth2 : powerlib/Elements/Series RLC Branch  LConnTagsString=__new0  RConnTagsString=__new0  BranchType=C  Resistance=0  Inductance=1e-3  SetiL0=off  InitialCurrent=0  Capacitance=y4*Cth2  Setx0=on  InitialVoltage=T2_initial_left  Measurements=Branch voltage
      settings: SourceProductName=Simscape Electrical
  Conn1 : PMIOPort  Side=Right
  wires:
  In1/1 -> Disp_Function/1, V3/1
  connections:
  x5*Rth2/LConn1 -- x4*Rth2/RConn1 -- y3*Cth2/LConn1
  x6*Rth2/LConn1 -- x5*Rth2/RConn1 -- y4*Cth2/LConn1
  x4*Rth2/LConn1 -- x4_g*Rth2_g/LConn1 -- V3/RConn1
  x6*Rth2/RConn1 -- x5_g*Rth2_g/RConn1 -- Conn1/RConn1
  Ground10/LConn1 -- y3*Cth2/RConn1
  y3_g*Cth2_g/LConn1 -- x4_g*Rth2_g/RConn1 -- x5_g*Rth2_g/LConn1
  Ground23/LConn1 -- y3_g*Cth2_g/RConn1
  Ground9/LConn1 -- y4*Cth2/RConn1
  Ground17/LConn1 -- V3/LConn1

== system Wall_Model_Version_1_8_2018a/ROOM/Qhuman ==
  "No_Male " : Inport
  No_Female : Inport  Port=2
  Ground3 : powerlib/Elements/Ground  LConnTagsString=a
      settings: SourceProductName=Simscape Electrical
  Heat_produced : M-S-Function  FunctionName=human
  I : powerlib/Electrical Sources/Controlled Current Source  Initialize=on  Source_Type=AC  Amplitude=1  Phase=0  Frequency=0  Measurements=None
      settings: SourceProductName=Simscape Electrical
  Conn1 : PMIOPort  Side=Right
  wires:
  "No_Male "/1 -> Heat_produced/1
  Heat_produced/1 -> I/1
  No_Female/1 -> Heat_produced/2
  connections:
  I/LConn1 -- Ground3/LConn1
  I/RConn1 -- Conn1/RConn1

== system Wall_Model_Version_1_8_2018a/ROOM/Qhvac ==
  Setpoint : Inport
  Tbs : Inport  Port=2
  Ground3 : powerlib/Elements/Ground  LConnTagsString=a
      settings: SourceProductName=Simscape Electrical
  I : powerlib/Electrical Sources/Controlled Current Source  Initialize=on  Source_Type=DC  Amplitude=5000  Phase=0  Frequency=0  Measurements=None
      settings: SourceProductName=Simscape Electrical
  PID Controller : simulink/Continuous/PID Controller  Controller=PI  Form=Parallel  TimeDomain=Continuous-time  SampleTime=-1  IntegratorMethod=Backward Euler  FilterMethod=Forward Euler  ControllerParametersSource=internal  P=0  I=101.417145566816  D=-296662.911304383  UseFilter=on  N=0.0135323447314473  TunerSelectOption=Transfer Function Based (PID Tuner App)  InitialConditionSource=internal  InitialConditionForIntegrator=22  InitialConditionForFilter=0  DifferentiatorICPrevScaledInput=0  ExternalReset=none  TrackingMode=off  Kt=1  LimitOutput=off  UpperSaturationLimit=0  LowerSaturationLimit=-15000  LinearizeAsGain=on  AntiWindupMode=none  Kb=1  POutMin=[]  POutMax=[]  IOutMin=[]  IOutMax=[]  DOutMin=[]  DOutMax=[]  NOutMin=[]  NOutMax=[]  SumOutMin=[]  SumOutMax=[]  SaturationOutMin=[]  SaturationOutMax=[]  PParamMin=[]  PParamMax=[]  IParamMin=[]  IParamMax=[]  DParamMin=[]  DParamMax=[]  NParamMin=[]  NParamMax=[]  KbParamMin=[]  KbParamMax=[]  KtParamMin=[]  KtParamMax=[]  KbOutMin=[]  KbOutMax=[]  KtOutMin=[]  KtOutMax=[]  IntegratorOutMin=[]  IntegratorOutMax=[]  FilterOutMin=[]  FilterOutMax=[]  SumI1OutMin=[]  SumI1OutMax=[]  SumI2OutMin=[]  SumI2OutMax=[]  SumI3OutMin=[]  SumI3OutMax=[]  SumI4OutMin=[]  SumI4OutMax=[]  SumDOutMin=[]  SumDOutMax=[]  DifferentiatorOutMin=[]  DifferentiatorOutMax=[]  FilterDiffOutCoefMin=[]  FilterDiffOutCoefMax=[]  ReciprocalOutMin=[]  ReciprocalOutMax=[]  SumDenOutMin=[]  SumDenOutMax=[]  SumNumOutMin=[]  SumNumOutMax=[]  DivideOutMin=[]  DivideOutMax=[]  IntegratorContinuousStateAttributes=''  IntegratorStateMustResolveToSignalObject=off  IntegratorRTWStateStorageClass=Auto  FilterContinuousStateAttributes=''  FilterStateMustResolveToSignalObject=off  FilterRTWStateStorageClass=Auto  ParallelPVariant=InternalParameters  IdealPVariant=Disabled  IVariant=InternalParameters  DVariant=Disabled  IntegratorVariant=Continuous  SatVariant=Disabled  AWVariant=Passthrough  PCopyVariant=Disabled  TRVariant=Disabled  FdbkBlocksVariant=Forward  IdealPFdbkVariant=Disabled  SatFdbkVariant=Disabled  DerivativeFilterVariant=Disabled  NVariant=Disabled  NCopyVariant=Disabled_SignalSpec  FilterICVariant=Disabled  IntegratorICVariant=InternalICs  ExternalResetVariant=Disabled  TRSumVariant=Passthrough  SumFdbkVariant=Disabled  SumVariant=Sum_PI
  Sum : Sum  Inputs=|+-
  Conn1 : PMIOPort  Side=Right
  Qhvac : Outport
  wires:
  PID Controller/1 -> I/1, Qhvac/1
  Setpoint/1 -> Sum/1
  Tbs/1 -> Sum/2
  Sum/1 -> PID Controller/1
  connections:
  I/RConn1 -- Conn1/RConn1
  I/LConn1 -- Ground3/LConn1

== system Wall_Model_Version_1_8_2018a/ROOM/Qlighting ==
  "No_light " : Inport
  Wattage : Inport  Port=2
  Ground3 : powerlib/Elements/Ground  LConnTagsString=a
      settings: SourceProductName=Simscape Electrical
  Heat_produced : M-S-Function  FunctionName=light1
  I : powerlib/Electrical Sources/Controlled Current Source  Initialize=on  Source_Type=AC  Amplitude=1  Phase=0  Frequency=0  Measurements=None
      settings: SourceProductName=Simscape Electrical
  Conn1 : PMIOPort  Side=Right
  wires:
  "No_light "/1 -> Heat_produced/1
  Heat_produced/1 -> I/1
  Wattage/1 -> Heat_produced/2
  connections:
  I/LConn1 -- Ground3/LConn1
  I/RConn1 -- Conn1/RConn1

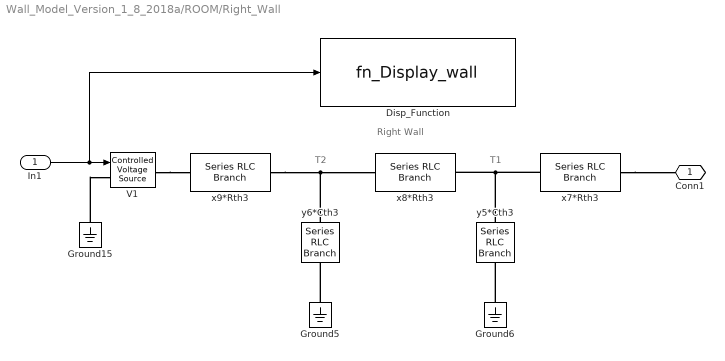
== system Wall_Model_Version_1_8_2018a/ROOM/Right_Wall ==
  note: Right Wall
  note: T2
  note: T1
  In1 : Inport
  Disp_Function : M-S-Function  FunctionName=fn_Display_wall
  Ground15 : powerlib/Elements/Ground  LConnTagsString=a
      settings: SourceProductName=Simscape Electrical
  Ground5 : powerlib/Elements/Ground  LConnTagsString=a
      settings: SourceProductName=Simscape Electrical
  Ground6 : powerlib/Elements/Ground  LConnTagsString=a
      settings: SourceProductName=Simscape Electrical
  V1 : powerlib/Electrical Sources/Controlled Voltage Source  Initialize=on  Source_Type=AC  Amplitude=0  Phase=0  Frequency=0  Measurements=None
      settings: SourceProductName=Simscape Electrical
  x7*Rth3 : powerlib/Elements/Series RLC Branch  LConnTagsString=__new0  RConnTagsString=__new0  BranchType=R  Resistance=x7*Rth3  Inductance=1e-3  SetiL0=off  InitialCurrent=0  Capacitance=1e-6  Setx0=off  InitialVoltage=0  Measurements=None
      settings: SourceProductName=Simscape Electrical
  x8*Rth3 : powerlib/Elements/Series RLC Branch  LConnTagsString=__new0  RConnTagsString=__new0  BranchType=R  Resistance=x8*Rth3  Inductance=1e-3  SetiL0=off  InitialCurrent=0  Capacitance=1e-6  Setx0=off  InitialVoltage=0  Measurements=None
      settings: SourceProductName=Simscape Electrical
  x9*Rth3 : powerlib/Elements/Series RLC Branch  LConnTagsString=__new0  RConnTagsString=__new0  BranchType=R  Resistance=x9*Rth3  Inductance=1e-3  SetiL0=off  InitialCurrent=0  Capacitance=1e-6  Setx0=off  InitialVoltage=0  Measurements=None
      settings: SourceProductName=Simscape Electrical
  y5*Cth3 : powerlib/Elements/Series RLC Branch  LConnTagsString=__new0  RConnTagsString=__new0  BranchType=C  Resistance=0  Inductance=1e-3  SetiL0=off  InitialCurrent=0  Capacitance=y5*Cth3  Setx0=on  InitialVoltage=T1_initial_right  Measurements=Branch voltage
      settings: SourceProductName=Simscape Electrical
  y6*Cth3 : powerlib/Elements/Series RLC Branch  LConnTagsString=__new0  RConnTagsString=__new0  BranchType=C  Resistance=0  Inductance=1e-3  SetiL0=off  InitialCurrent=0  Capacitance=y6*Cth3  Setx0=on  InitialVoltage=T2_initial_right  Measurements=Branch voltage
      settings: SourceProductName=Simscape Electrical
  Conn1 : PMIOPort  Side=Right
  wires:
  In1/1 -> Disp_Function/1, V1/1
  connections:
  x7*Rth3/RConn1 -- Conn1/RConn1
  x7*Rth3/LConn1 -- y5*Cth3/LConn1 -- x8*Rth3/RConn1
  y6*Cth3/LConn1 -- x9*Rth3/RConn1 -- x8*Rth3/LConn1
  Ground15/LConn1 -- V1/LConn1
  Ground5/LConn1 -- y6*Cth3/RConn1
  Ground6/LConn1 -- y5*Cth3/RConn1
  V1/RConn1 -- x9*Rth3/LConn1

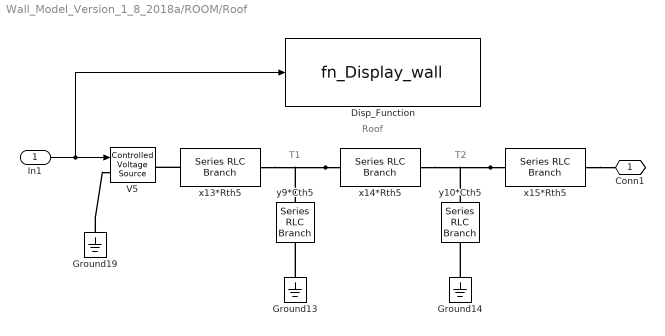
== system Wall_Model_Version_1_8_2018a/ROOM/Roof ==
  note: T1
  note: T2
  note: Roof
  In1 : Inport
  Disp_Function : M-S-Function  FunctionName=fn_Display_wall
  Ground13 : powerlib/Elements/Ground  LConnTagsString=a
      settings: SourceProductName=Simscape Electrical
  Ground14 : powerlib/Elements/Ground  LConnTagsString=a
      settings: SourceProductName=Simscape Electrical
  Ground19 : powerlib/Elements/Ground  LConnTagsString=a
      settings: SourceProductName=Simscape Electrical
  V5 : powerlib/Electrical Sources/Controlled Voltage Source  Initialize=on  Source_Type=AC  Amplitude=0  Phase=0  Frequency=0  Measurements=None
      settings: SourceProductName=Simscape Electrical
  x13*Rth5 : powerlib/Elements/Series RLC Branch  LConnTagsString=__new0  RConnTagsString=__new0  BranchType=R  Resistance=x13*Rth5  Inductance=1e-3  SetiL0=off  InitialCurrent=0  Capacitance=1e-6  Setx0=off  InitialVoltage=0  Measurements=None
      settings: SourceProductName=Simscape Electrical
  x14*Rth5 : powerlib/Elements/Series RLC Branch  LConnTagsString=__new0  RConnTagsString=__new0  BranchType=R  Resistance=x14*Rth5  Inductance=1e-3  SetiL0=off  InitialCurrent=0  Capacitance=1e-6  Setx0=off  InitialVoltage=0  Measurements=None
      settings: SourceProductName=Simscape Electrical
  x15*Rth5 : powerlib/Elements/Series RLC Branch  LConnTagsString=__new0  RConnTagsString=__new0  BranchType=R  Resistance=x15*Rth5  Inductance=1e-3  SetiL0=off  InitialCurrent=0  Capacitance=1e-6  Setx0=off  InitialVoltage=0  Measurements=None
      settings: SourceProductName=Simscape Electrical
  y10*Cth5 : powerlib/Elements/Series RLC Branch  LConnTagsString=__new0  RConnTagsString=__new0  BranchType=C  Resistance=0  Inductance=1e-3  SetiL0=off  InitialCurrent=0  Capacitance=y10*Cth5  Setx0=on  InitialVoltage=T2_initial_roof  Measurements=Branch voltage
      settings: SourceProductName=Simscape Electrical
  y9*Cth5 : powerlib/Elements/Series RLC Branch  LConnTagsString=__new0  RConnTagsString=__new0  BranchType=C  Resistance=0  Inductance=1e-3  SetiL0=off  InitialCurrent=0  Capacitance=y9*Cth5  Setx0=on  InitialVoltage=T1_initial_roof  Measurements=Branch voltage
      settings: SourceProductName=Simscape Electrical
  Conn1 : PMIOPort  Side=Right
  wires:
  In1/1 -> Disp_Function/1, V5/1
  connections:
  Ground14/LConn1 -- y10*Cth5/RConn1
  x15*Rth5/RConn1 -- Conn1/RConn1
  x14*Rth5/LConn1 -- x13*Rth5/RConn1 -- y9*Cth5/LConn1
  x15*Rth5/LConn1 -- x14*Rth5/RConn1 -- y10*Cth5/LConn1
  Ground19/LConn1 -- V5/LConn1
  x13*Rth5/LConn1 -- V5/RConn1
  Ground13/LConn1 -- y9*Cth5/RConn1

== system Wall_Model_Version_1_8_2018a/ROOM/Room ==
  In1 : Inport
  Disp_Function : M-S-Function  FunctionName=fn_Display_wall
  wires:
  In1/1 -> Disp_Function/1

== matlab function Wall_Model_Version_1_8_2018a/ROOM/IEQ_INDEX/IAQ_CO2 ==
  data: C input; IAQ_CO2 output
function IAQ_CO2 = fcn(C)
% C in PPM measured 8 hr average
% IAQ
 C_hi = 0; C_lo = 0; I_hi = 0; I_lo = 0;

% Good
if C<400

elseif 400<=C && C<700
    C_hi = 699; C_lo = 400; I_hi = 50; I_lo = 0;
% Moderate
elseif 700<=C && C<1000
    C_hi = 999; C_lo = 700; I_hi = 100; I_lo = 51;
% Unhealthy
elseif 1000<=C && C<1500
    C_hi = 1499; C_lo = 1000; I_hi = 200; I_lo = 101;    
% Very Unhealthy
elseif 1500<=C && C<4500
    C_hi = 4499; C_lo = 1500; I_hi = 300; I_lo = 201;
% Emergency
elseif 4500<=C %&& C<20000
    C_hi = 20000; C_lo = 4500; I_hi = 500; I_lo = 301;    
end

IAQ_CO2 = (((I_hi - I_lo)*(C - C_lo))/(C_hi - C_lo)) + I_lo;

== matlab function Wall_Model_Version_1_8_2018a/ROOM/IEQ_INDEX/IAQ_CO ==
  data: C input; IAQ_CO output
function IAQ_CO = fcn(C)
% C in PPM measured 8 hr average
% IAQ
 C_hi = 0; C_lo = 0; I_hi = 0; I_lo = 0;
 
% Good
if 0<=C && C<5
    C_hi = 4.99; C_lo = 0; I_hi = 50; I_lo = 0;
% Moderate
elseif 5<=C && C<9
    C_hi = 8.99; C_lo = 5; I_hi = 100; I_lo = 51;
% Unhealthy
elseif 9<=C && C<15
    C_hi = 14.99; C_lo = 9; I_hi = 200; I_lo = 101;    
% Very Unhealthy
elseif 15<=C && C<30
    C_hi = 29.99; C_lo = 15; I_hi = 300; I_lo = 201;
% Emergency
elseif 30<=C %&& C<2000
    C_hi = 2000; C_lo = 30; I_hi = 500; I_lo = 301;    
end


IAQ_CO = (((I_hi - I_lo)*(C - C_lo))/(C_hi - C_lo)) + I_lo;

== matlab function Wall_Model_Version_1_8_2018a/ROOM/IEQ_INDEX/IAQ_O3 ==
  data: C input; IAQ_O3 output
function IAQ_O3 = fcn(C)
% C in PPB measured 8 hr average
% IAQ
 C_hi = 0; C_lo = 0; I_hi = 0; I_lo = 0;

% Good
if 0<=C && C<50
    C_hi = 49.9; C_lo = 0; I_hi = 50; I_lo = 0;
% Moderate
elseif 50<=C && C<70
    C_hi = 69.9; C_lo = 50; I_hi = 100; I_lo = 51;
% Unhealthy
elseif 70<=C && C<100
    C_hi = 99.9; C_lo = 70; I_hi = 200; I_lo = 101;    
% Very Unhealthy
elseif 100<=C && C<200
    C_hi = 199.9; C_lo = 100; I_hi = 300; I_lo = 201;
% Emergency
elseif 200<=C %&& C<700
    C_hi = 700; C_lo = 200; I_hi = 500; I_lo = 301;    
end

IAQ_O3 = (((I_hi - I_lo)*(C - C_lo))/(C_hi - C_lo)) + I_lo;

== matlab function Wall_Model_Version_1_8_2018a/ROOM/IEQ_INDEX/IAQ_HCHO ==
  data: C input; IAQ_HCHO output
function IAQ_HCHO = fcn(C)
% C in mg/m3 measured 8 hr average
% IAQ
% reference : https://www.ncbi.nlm.nih.gov/pmc/articles/PMC3175005/
 C_hi = 0; C_lo = 0; I_hi = 0; I_lo = 0;

% Good
if 0<=C && C<0.05
    C_hi = 0.05; C_lo = 0; I_hi = 50; I_lo = 0;
% Moderate
elseif 0.05<=C && C<0.12
    C_hi = 0.119; C_lo = 0.05; I_hi = 100; I_lo = 51;
% Unhealthy
elseif 0.12<=C && C<0.25
    C_hi = 0.249; C_lo =0.12; I_hi = 200; I_lo = 101;    
% Very Unhealthy
elseif 0.25<=C && C<0.6
    C_hi = 0.59; C_lo = 0.25; I_hi = 300; I_lo = 201;
% Emergency
elseif 0.6<=C %&& C<2.5
    C_hi = 2.5; C_lo = 0.6; I_hi = 500; I_lo = 301;    
end

IAQ_HCHO = (((I_hi - I_lo)*(C - C_lo))/(C_hi - C_lo)) + I_lo;

== matlab function Wall_Model_Version_1_8_2018a/ROOM/IEQ_INDEX/IAQ_VOC ==
  data: C input; IAQ_VOC output
function IAQ_VOC = fcn(C)
% C in ppm measured 8 hr average
% IAQ
% reference :THE A DETAILED STUDY OF VOLATILE ORGANIC COMPOUNDS
% OF 5 AIR-CONDITIONED BUILDINGS IN SINGAPORE
% Residential Indoor Air Quality Guideline TOLUENE
 C_hi = 0; C_lo = 0; I_hi = 0; I_lo = 0;

% Good
if 0<=C && C<1.2
    C_hi = 1.19; C_lo = 0; I_hi = 50; I_lo = 0;
% Moderate
elseif 1.2<=C && C<2
    C_hi = 0.119; C_lo = 0.05; I_hi = 100; I_lo = 51;
% Unhealthy
elseif 2<=C && C<3
    C_hi = 2.99; C_lo =2; I_hi = 200; I_lo = 101;    
% Very Unhealthy
elseif 3<=C && C<4
    C_hi = 3.99; C_lo = 3; I_hi = 300; I_lo = 201;
% Emergency
elseif 4<=C %&& C<6
    C_hi = 6; C_lo = 4; I_hi = 500; I_lo = 301;    
end

IAQ_VOC = (((I_hi - I_lo)*(C - C_lo))/(C_hi - C_lo)) + I_lo;

== matlab function Wall_Model_Version_1_8_2018a/ROOM/IEQ_INDEX/IAQ_PM2_5 ==
  data: C input; IAQ_PM2_5 output
function IAQ_PM2_5 = fcn(C)
% C in UG/M3 measured 8 hr average
% IAQ
% reference :THE A DETAILED STUDY OF VOLATILE ORGANIC COMPOUNDS
% OF 5 AIR-CONDITIONED BUILDINGS IN SINGAPORE 
 C_hi = 0; C_lo = 0; I_hi = 0; I_lo = 0;

% Good
if 0<=C && C<10
    C_hi = 9.9; C_lo = 0; I_hi = 50; I_lo = 0;
% Moderate
elseif 10<=C && C<40
    C_hi = 39.9; C_lo = 10; I_hi = 100; I_lo = 51;
% Unhealthy
elseif 40<=C && C<130
    C_hi = 129.9; C_lo = 40; I_hi = 200; I_lo = 101;    
% Very Unhealthy
elseif 130<=C && C<250
    C_hi = 249.9; C_lo = 130; I_hi = 300; I_lo = 201;
% Emergency
elseif 250<=C %&& C<500
    C_hi = 500; C_lo = 250; I_hi = 500; I_lo = 301;    
end

IAQ_PM2_5 = (((I_hi - I_lo)*(C - C_lo))/(C_hi - C_lo)) + I_lo;

== matlab function Wall_Model_Version_1_8_2018a/ROOM/IEQ_INDEX/IAQ_PM10 ==
  data: C input; IAQ_PM10 output
function IAQ_PM10 = fcn(C)
% C in UG/M3 measured 8 hr average
% IAQ
% reference :BCA, SINGAPORE 
 C_hi = 0; C_lo = 0; I_hi = 0; I_lo = 0;

% Good
if 0<=C && C<50
    C_hi = 49.9; C_lo = 0; I_hi = 50; I_lo = 0;
% Moderate
elseif 50<=C && C<150
    C_hi = 149.9; C_lo = 50; I_hi = 100; I_lo = 51;
% Unhealthy
elseif 150<=C && C<350
    C_hi = 349.9; C_lo = 150; I_hi = 200; I_lo = 101;    
% Very Unhealthy
elseif 350<=C && C<425
    C_hi = 424.9; C_lo = 350; I_hi = 300; I_lo = 201;
% Emergency
elseif 425<=C %&& C<600
    C_hi = 600; C_lo = 250; I_hi = 500; I_lo = 301;    
end

IAQ_PM10 = (((I_hi - I_lo)*(C - C_lo))/(C_hi - C_lo)) + I_lo;

== matlab function Wall_Model_Version_1_8_2018a/DISPLAY1/IAQ_CO ==
  data: C input; IAQ_CO output
function IAQ_CO = fcn(C)
% C in PPM measured 8 hr average
% IAQ
 C_hi = 0; C_lo = 0; I_hi = 0; I_lo = 0;
 
% Good
if 0<=C && C<5
    C_hi = 4.99; C_lo = 0; I_hi = 50; I_lo = 0;
% Moderate
elseif 5<=C && C<9
    C_hi = 8.99; C_lo = 5; I_hi = 100; I_lo = 51;
% Unhealthy
elseif 9<=C && C<15
    C_hi = 14.99; C_lo = 9; I_hi = 200; I_lo = 101;    
% Very Unhealthy
elseif 15<=C && C<30
    C_hi = 29.99; C_lo = 15; I_hi = 300; I_lo = 201;
% Emergency
elseif 30<=C %&& C<2000
    C_hi = 2000; C_lo = 30; I_hi = 500; I_lo = 301;    
end


IAQ_CO = (((I_hi - I_lo)*(C - C_lo))/(C_hi - C_lo)) + I_lo;

== matlab function Wall_Model_Version_1_8_2018a/DISPLAY1/IAQ_CO2 ==
  data: C input; IAQ_CO2 output
function IAQ_CO2 = fcn(C)
% C in PPM measured 8 hr average
% IAQ
 C_hi = 0; C_lo = 0; I_hi = 0; I_lo = 0;

% Good
if C<400

elseif 400<=C && C<700
    C_hi = 699; C_lo = 400; I_hi = 50; I_lo = 0;
% Moderate
elseif 700<=C && C<1000
    C_hi = 999; C_lo = 700; I_hi = 100; I_lo = 51;
% Unhealthy
elseif 1000<=C && C<1500
    C_hi = 1499; C_lo = 1000; I_hi = 200; I_lo = 101;    
% Very Unhealthy
elseif 1500<=C && C<4500
    C_hi = 4499; C_lo = 1500; I_hi = 300; I_lo = 201;
% Emergency
elseif 4500<=C %&& C<20000
    C_hi = 20000; C_lo = 4500; I_hi = 500; I_lo = 301;    
end

IAQ_CO2 = (((I_hi - I_lo)*(C - C_lo))/(C_hi - C_lo)) + I_lo;
